simulink model "Question2"  (R2017a)
settings: Solver=FixedStepAuto  StartTime=0.0  StopTime=25  FixedStep=0.05  RelTol=1e-3
undefined symbols (not defined in the file): n1, n2, y1i, y2i
settings Model: Creator=Faizan Tariq  LastModifiedBy=Faizan Tariq

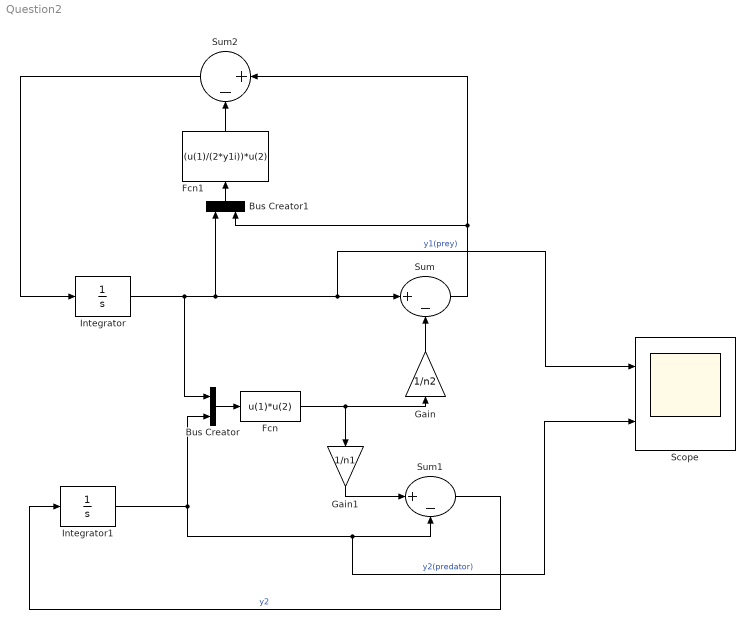
== system Question2 ==
  Bus Creator : BusCreator  Inputs=2
  Bus Creator1 : BusCreator  Inputs=2
  Fcn : Fcn  Expr=u(1)*u(2)
  Fcn1 : Fcn  Expr=(u(1)/(2*y1i))*u(2)
  Gain : Gain  Gain=1/n2
  Gain1 : Gain  Gain=1/n1
  Integrator : Integrator  InitialCondition=y1i
  Integrator1 : Integrator  InitialCondition=y2i
  Scope : Scope  NumInputPorts=2
  Sum : Sum  Inputs=|+-
  Sum1 : Sum  Inputs=|+-
  Sum2 : Sum  Inputs=|+-
  wires:
  Integrator/1 -> Bus Creator/1, Bus Creator1/1, Scope/1, Sum/1  "y1(prey)"
  Gain/1 -> Sum/2
  Bus Creator/1 -> Fcn/1
  Integrator1/1 -> Scope/2, Sum1/2, Bus Creator/2  "y2(predator)"
  Fcn/1 -> Gain1/1, Gain/1
  Sum1/1 -> Integrator1/1  "y2"
  Gain1/1 -> Sum1/1
  Sum/1 -> Sum2/1, Bus Creator1/2
  Sum2/1 -> Integrator/1
  Fcn1/1 -> Sum2/2
  Bus Creator1/1 -> Fcn1/1
